simulink model "system_model_2"  (R2021a)
settings: Solver=VariableStepAuto  StartTime=0.0  StopTime=3000  RelTol=1e-3
values from neighbouring files (symbols this model uses):
  alpha = 0.3    [backup.m]    (also in tf_estimate.m = 0.1)
  D_active = 0    [tf_estimate.m]
  den = sys.Denominator    [backup.m]    (also in tf_estimate.m)
  I_active = 1    [tf_estimate.m]
  kp = 1/mag(1,1,min(k))    [backup.m]    (also in tf_estimate.m = 1/mag(k))
  num = sys.Numerator    [backup.m]    (also in tf_estimate.m)
  set_temp = 200 - temp(1)    [tf_estimate.m]
  td = 1/(wc*sqrt(alpha))    [backup.m]    (also in tf_estimate.m)
  temp = fscanf(fileID,formatSpec,sizeA)    [backup.m]    (also in tf_estimate.m)
  ti = Ni*1/wc    [backup.m]    (also in tf_estimate.m)
settings Model: Creator=leouh  LastModifiedBy=leouh

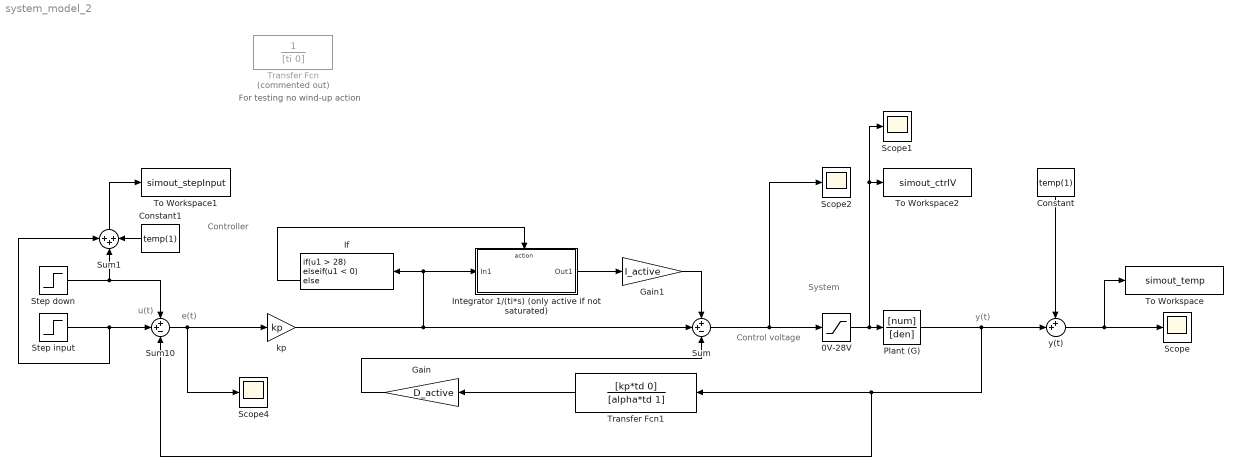
== system system_model_2 ==
  note: For testing no wind-up action
  note: Controller
  note: e(t)
  note: y(t)
  note: u(t)
  note: Control voltage
  note: System
  0V-28V : Saturate  UpperLimit=28  LowerLimit=0  ZeroCross=off
  Constant : Constant  Value=temp(1)
  Constant1 : Constant  Value=temp(1)
  Gain : Gain  Gain=D_active
  Gain1 : Gain  Gain=I_active
  If : If  IfExpression=u1 > 28  ElseIfExpressions=u1 < 0  ZeroCross=off
  Integrator 1/(ti*s) (only active if not saturated) : Subsystem  TreatAsAtomicUnit=on
  Plant (G) : TransferFcn  Numerator=[num]  Denominator=[den]
  Scope{,1..2,4} (4 alike) : Scope
  Step down : Step  Time=2000  After=-30  SampleTime=0
  Step input : Step  After=set_temp  SampleTime=0
  Sum : Sum  Inputs=++-
  Sum1 : Sum  Inputs=+++
  Sum10 : Sum  Inputs=++-
  To Workspace : ToWorkspace  VariableName=simout_temp  SaveFormat=Timeseries  SampleTime=-1
  To Workspace1 : ToWorkspace  VariableName=simout_stepInput  SaveFormat=Timeseries  SampleTime=-1
  To Workspace2 : ToWorkspace  VariableName=simout_ctrlV  SaveFormat=Timeseries  SampleTime=-1
  Transfer Fcn : TransferFcn  Commented=on  Denominator=[ti 0]
  Transfer Fcn1 : TransferFcn  Numerator=[kp*td 0]  Denominator=[alpha*td 1]
  kp : Gain  Gain=kp
  y(t) : Sum  Inputs=++|
  wires:
  Constant/1 -> y(t)/1
  Step input/1 -> Sum1/1, Sum10/2
  Step down/1 -> Sum10/1, Sum1/2
  y(t)/1 -> To Workspace/1, Scope/1
  Sum10/1 -> Scope4/1, kp/1
  Sum/1 -> 0V-28V/1, Scope2/1
  0V-28V/1 -> Scope1/1, To Workspace2/1, Plant (G)/1
  Plant (G)/1 -> Sum10/3, Transfer Fcn1/1, y(t)/2
  Transfer Fcn1/1 -> Gain/1
  Sum1/1 -> To Workspace1/1
  Constant1/1 -> Sum1/3
  Gain/1 -> Sum/3
  If/3 -> Integrator 1/(ti*s) (only active if not saturated)/Action
  kp/1 -> Sum/2, If/1, Integrator 1/(ti*s) (only active if not saturated)/1(In1)
  Integrator 1/(ti*s) (only active if not saturated)/1(Out1) -> Gain1/1
  Gain1/1 -> Sum/1

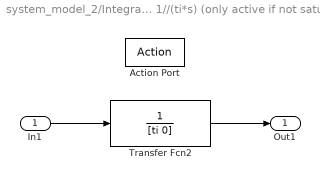
== system system_model_2/Integrator 1//(ti*s) (only active if not saturated) ==
  In1 : Inport
  Action Port : ActionPort  ActionPortLabel=else
  Transfer Fcn2 : TransferFcn  Denominator=[ti 0]
  Out1 : Outport
  wires:
  In1/1 -> Transfer Fcn2/1
  Transfer Fcn2/1 -> Out1/1
